simulink model "trqv"  (R2022b)
settings: Solver=VariableStepAuto  StartTime=0.0  StopTime=10.0  RelTol=1e-3
values from neighbouring files (symbols this model uses):
  Caf = 460    [trqvparameter.m]
  Car = 440    [trqvparameter.m]
  lf = 0.761    [trqvparameter.m]
  lr = 0.831    [trqvparameter.m]
  m = 340    [trqvparameter.m]
settings Model: Creator=12045  LastModifiedBy=12045

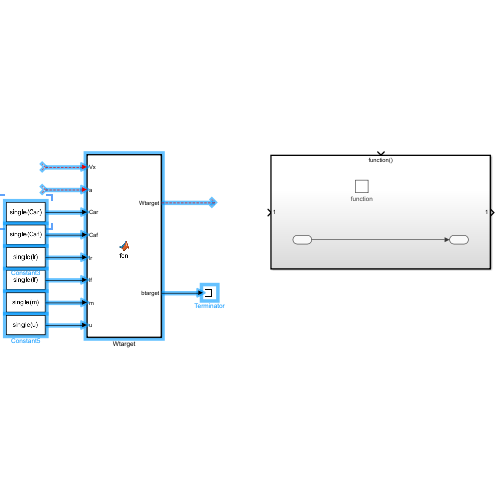
[thumbnail: Simulink's stored preview of the top-level diagram]
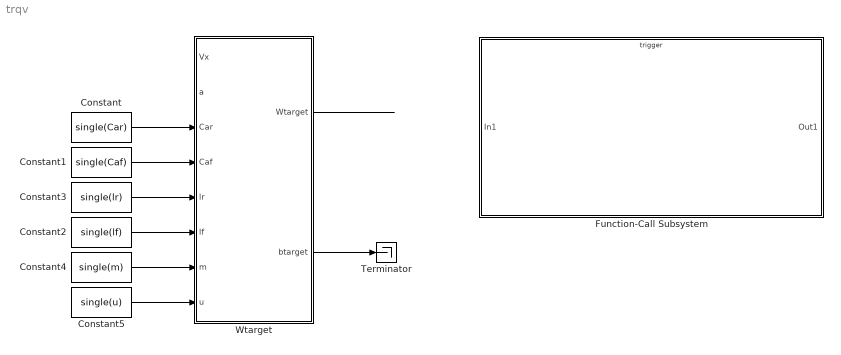
== system trqv ==
  Constant : Constant  Value=single(Car)
  Constant1 : Constant  Value=single(Caf)
  Constant2 : Constant  Value=single(lf)
  Constant3 : Constant  Value=single(lr)
  Constant4 : Constant  Value=single(m)
  Constant5 : Constant  Value=single(u)
  Function-Call Subsystem : Subsystem  TreatAsAtomicUnit=on
  Terminator : Terminator
  Wtarget : MATLAB Function  TreatAsAtomicUnit=on
  wires:
  Constant/1 -> Wtarget/3(Car)
  Constant1/1 -> Wtarget/4(Caf)
  Constant2/1 -> Wtarget/6(lf)
  Constant3/1 -> Wtarget/5(lr)
  Constant4/1 -> Wtarget/7(m)
  Constant5/1 -> Wtarget/8(u)
  ? -> Wtarget/1(Vx)
  ? -> Wtarget/2(a)
  Wtarget/2(btarget) -> Terminator/1
  Wtarget/1(Wtarget) -> ?

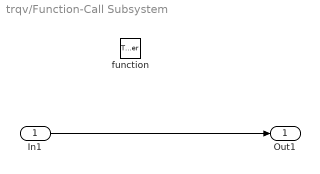
== system trqv/Function-Call Subsystem ==
  In1 : Inport
  function : TriggerPort  TriggerType=function-call  VariantControl=(inherit)
  Out1 : Outport
  wires:
  In1/1 -> Out1/1

== matlab function trqv/Wtarget ==
  data: Vx input size=1; Wtarget output size=1; a input size=1; Car input size=1; Caf input size=1; lr input size=1; lf input size=1; m input; u input; btarget output
function [Wtarget,btarget] = fcn(Vx,a,Car,Caf,lr,lf,m,u)
Wdes = Vx*a/(lf+lr+(m*Vx*Vx*(lr*Car-lf*Caf)/Caf/Car/(lr+lf)/2));
Wu = 0.85*u*9.8/Vx;
if abs(Wdes)<=Wu
Wtarget = Wdes;
else
    Wtarget = Wu*sign(Wdes);
end
bdes = (lr-lf*m*Vx*Vx/Car/(lf+lr)/2)*a/(lr+lf+m*Vx*Vx*(lr*Car-lf*Caf)/Car/Caf/(lf+lr)/2);
bu = atan(0.02*u*9.8);
if abs(bdes)<=bu
btarget = bdes;
else
    btarget = bu*sign(bdes);
end
